simulink model "uz_6ph_pu_vsd_voltages_state_machine"  (R2021a)
settings: Solver=FixedStepDiscrete  StartTime=0.0  StopTime=3*t_ADC  RelTol=1e-3
values from neighbouring files (symbols this model uses):
  A = 1.0    (= 1)    [uz_6ph_pu_vsd_voltages_init.m]    (also in uz_mpc_6ph_init.m; uz_mpc_6ph_state_machine_init.m)
  f = n_rpm/60.0*p    (= 250)    [uz_6ph_pu_vsd_voltages_init.m]    (also in uz_mpc_6ph_init.m; uz_mpc_6ph_state_machine_init.m)
  t_ADC = 1/f_ADC    (= 1e-05)    [uz_6ph_pu_vsd_voltages_init.m]    (also in uz_mpc_6ph_init.m; uz_mpc_6ph_state_machine_init.m; uz_typeconv_init.m)
  t_clock = 1/f_clock    (= 1e-08)    [uz_6ph_pu_vsd_voltages_init.m]    (also in uz_mpc_6ph_init.m; uz_mpc_6ph_state_machine_init.m; uz_typeconv_init.m)
  v_dc = 565.0    (= 565)    [uz_6ph_pu_vsd_voltages_init.m]    (also in uz_mpc_6ph_init.m; uz_mpc_6ph_state_machine_init.m)
  VB = sqrt(2/3)*VR    [uz_6ph_pu_vsd_voltages_init.m]    (also in uz_mpc_6ph_init.m; uz_mpc_6ph_state_machine_init.m)
libraries: fl_lib x7, nesl_utility x7, simulink x3, hdlsllib x2, ee_lib x2
settings Model: DataTypeOverride=Off  Creator=micha  LastModifiedBy=micha
settings SolverCC: AlgebraicLoopSolver=TrustRegion
settings DataIOCC: LimitDataPoints=on  SaveOutput=off  SaveTime=off
settings OptimizationCC: BlockReduction=off  ConditionallyExecuteInputs=off  DefaultParameterBehavior=Inlined  LifeSpan=inf
settings DebuggingCC: AlgebraicLoopMsg=error  SingleTaskRateTransMsg=error  AllowSymbolicDim=off  StrictBusMsg=ErrorOnBusTreatedAsVector  SFUnexpectedBacktrackingDiag=warning  SFNoUnconditionalDefaultTransitionDiag=warning  SFExecutionAtInitializationDiag=none  SFMachineParentedDataDiag=warning  ArithmeticOperatorsInVariantConditions=warning
settings HardwareCC: ProdBitPerPointer=32  ProdBitPerSizeT=32  ProdBitPerPtrDiffT=32  ProdLargestAtomicFloat=None  ProdIntDivRoundTo=Undefined  ProdEndianess=Unspecified  ProdWordSize=32  ProdHWDeviceType=ASIC/FPGA->ASIC/FPGA  ProdEqTarget=off
settings SFSimCC: SimUseLocalCustomCode=off  CustomCodeUndefinedFunction=UseInterfaceOnly
settings RTWCC: RTWUseLocalCustomCode=off
settings CodeAppCC: StateflowObjectComments=on
settings GRTTargetCC: TargetLangStandard=C89/C90 (ANSI)
settings ConfigComp: CovScope=ReferencedModels  CovMetricSettings=dw  CovSaveCumulativeToWorkspaceVar=on  CovSaveSingleToWorkspaceVar=on  CovExternalEMLEnable=off  CovSFcnEnable=off

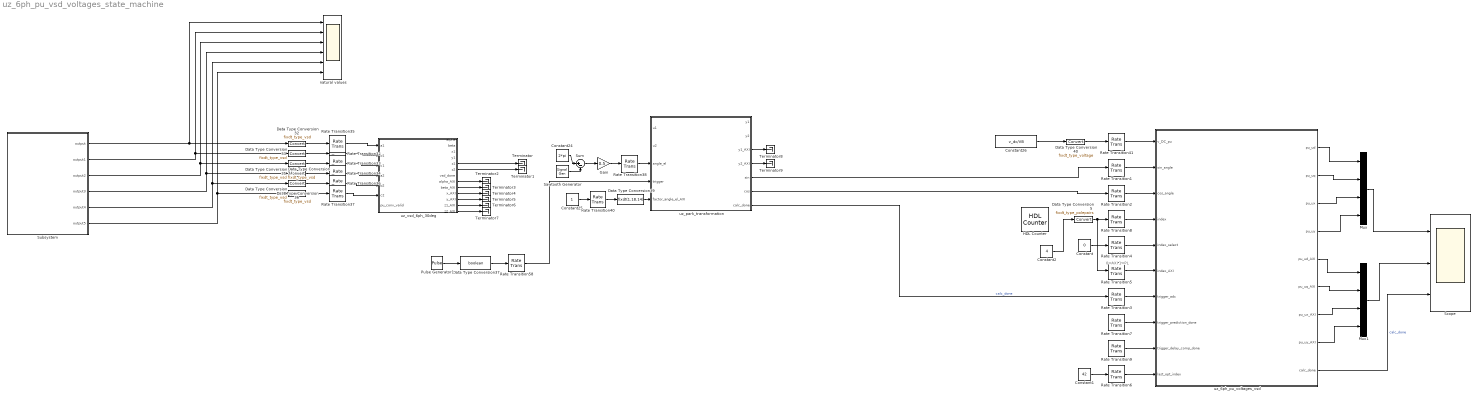
== system uz_6ph_pu_vsd_voltages_state_machine ==
  note: 0=AXI 1=PL
  Constant : Constant  Value=0  OutDataTypeStr=boolean
  Constant1 : Constant  Value=42  OutDataTypeStr=uint32
  Constant2 : Constant  Value=4  OutDataTypeStr=uint32
  Constant24 : Constant  Value=2*pi
  Constant25 : Constant
  Constant26 : Constant  Value=v_dc/VB
  Data Type Conversion{32..36,38} (6 alike) : DataTypeConversion  OutDataTypeStr=fixdt_type_vsd
  Data Type Conversion37 : DataTypeConversion  OutDataTypeStr=boolean
  Data Type Conversion39 : DataTypeConversion  OutDataTypeStr=fixdt(1,18,14)
  Data Type Conversion40 : DataTypeConversion  OutDataTypeStr=fixdt_type_voltage
  Data Type Conversion5 : DataTypeConversion  OutDataTypeStr=fixdt_type_polepairs
  Gain : Gain  Gain=0.5
  HDL Counter : hdlsllib/Sources/HDL Counter  CountType=Count limited  CountInit=1  CountStep=1  CountMax=64  CountFromType=Initial value  CountFrom=1  CountResetPort=off  CountLoadPort=off  CountEnbPort=off  CountDirPort=off  CountHitOutputPort=off  CountDataType=Unsigned  CountWordLen=8  CountFracLen=0  CountSampTime=t_ADC
  Mux : Mux
  Mux1 : Mux
  Pulse Generator1 : DiscretePulseGenerator  PulseType=Time based  Period=t_ADC  PulseWidth=5
  Rate Transition{1..2,4,32..38,40..41,58} (13 alike) : RateTransition  OutPortSampleTime=t_clock
  Rate Transition{3,5..9} (6 alike) : RateTransition  InitialCondition=1  OutPortSampleTime=t_clock
  Sawtooth Generator : SignalGenerator  WaveForm=sawtooth  Amplitude=2*pi  Frequency=2*pi*f  Units=rad/sec
  Scope : Scope  NumInputPorts=3
  Subsystem : Subsystem
  Sum : Sum  Inputs=|+-
  Terminator{,1..9} (10 alike) : Terminator
  natural values : Scope  NumInputPorts=6
  uz_6ph_pu_voltages_vsd : Subsystem  TreatAsAtomicUnit=on
  uz_park_transformation : Subsystem  TreatAsAtomicUnit=on
  uz_vsd_6ph_30deg : Subsystem  TreatAsAtomicUnit=on
  wires:
  Data Type Conversion5/1 -> Rate Transition8/1, Rate Transition5/1
  Rate Transition8/1 -> uz_6ph_pu_voltages_vsd/4(index)
  Constant26/1 -> Data Type Conversion40/1
  Rate Transition41/1 -> uz_6ph_pu_voltages_vsd/1(v_DC_pu)
  Data Type Conversion40/1 -> Rate Transition41/1
  Data Type Conversion35/1 -> Rate Transition34/1
  uz_vsd_6ph_30deg/5(z1) -> Terminator/1
  Rate Transition40/1 -> Data Type Conversion39/1
  Sawtooth Generator/1 -> Sum/2
  Constant25/1 -> Rate Transition40/1
  Data Type Conversion34/1 -> Rate Transition33/1
  Gain/1 -> Rate Transition38/1
  Subsystem/4(output3) -> Data Type Conversion35/1, natural values/4
  Sum/1 -> Gain/1
  Subsystem/5(output4) -> Data Type Conversion36/1, natural values/5
  Rate Transition33/1 -> uz_vsd_6ph_30deg/3(c1)
  uz_vsd_6ph_30deg/9(beta_AXI) -> Terminator3/1
  Rate Transition34/1 -> uz_vsd_6ph_30deg/4(a2)
  Rate Transition37/1 -> uz_vsd_6ph_30deg/6(c2)
  uz_vsd_6ph_30deg/6(z2) -> Terminator1/1
  uz_vsd_6ph_30deg/10(x_AXI) -> Terminator4/1
  Data Type Conversion39/1 -> uz_park_transformation/5(factor_angle_el_AXI)
  Subsystem/3(output2) -> Data Type Conversion34/1, natural values/3
  Subsystem/2(output1) -> natural values/2, Data Type Conversion33/1
  Data Type Conversion38/1 -> Rate Transition37/1
  Data Type Conversion33/1 -> Rate Transition32/1
  Rate Transition35/1 -> uz_vsd_6ph_30deg/1(a1)
  Rate Transition36/1 -> uz_vsd_6ph_30deg/5(b2)
  Constant24/1 -> Sum/1
  Subsystem/1(output) -> natural values/1, Data Type Conversion32/1
  uz_vsd_6ph_30deg/11(y_AXI) -> Terminator5/1
  Subsystem/6(output5) -> natural values/6, Data Type Conversion38/1
  uz_park_transformation/3(y1_AXI) -> Terminator8/1
  Rate Transition32/1 -> uz_vsd_6ph_30deg/2(b1)
  uz_vsd_6ph_30deg/8(alpha_AXI) -> Terminator2/1
  Data Type Conversion36/1 -> Rate Transition36/1
  uz_vsd_6ph_30deg/12(z1_AXI) -> Terminator6/1
  uz_park_transformation/4(y2_AXI) -> Terminator9/1
  Data Type Conversion32/1 -> Rate Transition35/1
  uz_vsd_6ph_30deg/13(z2_AXI) -> Terminator7/1
  uz_park_transformation/5(sin) -> Rate Transition1/1
  uz_park_transformation/6(cos) -> Rate Transition2/1
  Rate Transition1/1 -> uz_6ph_pu_voltages_vsd/2(sin_angle)
  Rate Transition2/1 -> uz_6ph_pu_voltages_vsd/3(cos_angle)
  Data Type Conversion37/1 -> Rate Transition58/1
  Rate Transition58/1 -> uz_park_transformation/4(trigger)
  Pulse Generator1/1 -> Data Type Conversion37/1
  Rate Transition3/1 -> uz_6ph_pu_voltages_vsd/7(trigger_adc)
  uz_park_transformation/7(calc_done) -> Rate Transition3/1  "calc_done"
  uz_6ph_pu_voltages_vsd/1(pu_ud) -> Mux/1
  uz_6ph_pu_voltages_vsd/2(pu_uq) -> Mux/2
  uz_6ph_pu_voltages_vsd/3(pu_ux) -> Mux/3
  uz_6ph_pu_voltages_vsd/4(pu_uy) -> Mux/4
  Mux/1 -> Scope/1
  uz_6ph_pu_voltages_vsd/9(calc_done) -> Scope/3  "calc_done"
  Constant2/1 -> Data Type Conversion5/1
  Rate Transition38/1 -> uz_park_transformation/3(angle_el)
  Rate Transition4/1 -> uz_6ph_pu_voltages_vsd/5(index_select)
  Rate Transition5/1 -> uz_6ph_pu_voltages_vsd/6(index_AXI)
  Constant/1 -> Rate Transition4/1
  Mux1/1 -> Scope/2
  uz_6ph_pu_voltages_vsd/5(pu_ud_AXI) -> Mux1/1
  uz_6ph_pu_voltages_vsd/8(pu_uy_AXI) -> Mux1/4
  uz_6ph_pu_voltages_vsd/7(pu_ux_AXI) -> Mux1/3
  uz_6ph_pu_voltages_vsd/6(pu_uq_AXI) -> Mux1/2
  Rate Transition6/1 -> uz_6ph_pu_voltages_vsd/10(last_opt_index)
  Constant1/1 -> Rate Transition6/1
  Rate Transition7/1 -> uz_6ph_pu_voltages_vsd/8(trigger_prediction_done)
  Rate Transition9/1 -> uz_6ph_pu_voltages_vsd/9(trigger_delay_comp_done)

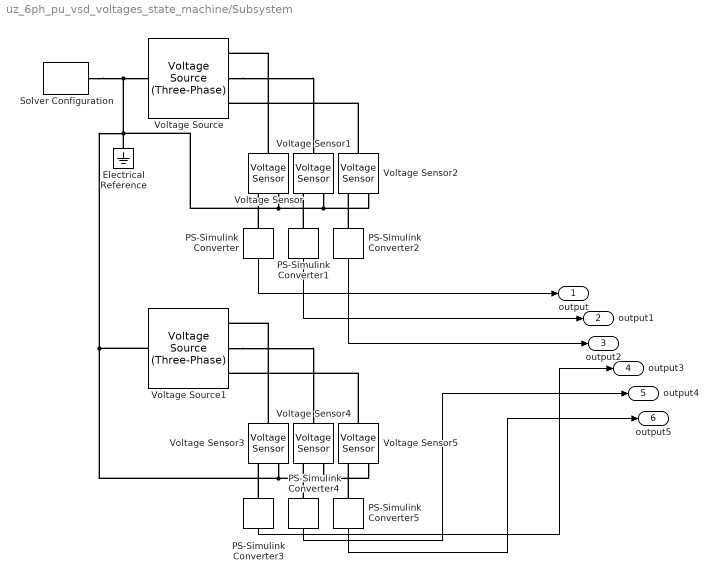
== system uz_6ph_pu_vsd_voltages_state_machine/Subsystem ==
  Electrical Reference : fl_lib/Electrical/Electrical Elements/Electrical Reference
  PS-Simulink Converter{,1..5} (6 alike) : nesl_utility/PS-Simulink Converter  PhysicalDomain=network_engine_domain  SubClassName=ps_output  LeftPortType=input  RightPortType=output  PseudoPeriodic=off  Frequencies=[]  Unit=1  AffineConversion=off
  Solver Configuration : nesl_utility/Solver Configuration  PhysicalDomain=network_engine_domain  SubClassName=solver  LeftPortType=input  RightPortType=generic  Tones=[]  Harmonics=[]  SimulateNoise=off  Profile=off  UseLocalSampling=off  EnableSwitchedLinearOptims=on  FrequencyDomain=off  UseCCode=off  RelTol=0.001  AbsTol=1e-06  MinStep=1e-09  ToWorkspace=off  RevertToSquareIcSolve=off  NumHomotopyIterations=100  PhasorMode=off  PhasorModeNumHarmonics=1  DoDC=off  ResidualTolerance=1e-09  UseLocalSolver=on  LocalSolverChoice=NE_BACKWARD_EULER_ADVANCER  LocalSolverSampleTime=1e-6  DoFixedCost=on  MaxNonlinIter=3  MaxModeIter=2  ComputeImpulses=off  ImpulseIterations=2  LinearAlgebra=Sparse  EquationFormulation=NE_TIME_EF  DelaysMemoryBudget=1024  AutomaticFiltering=on  FilteringTimeConstant=0.001  PartitionStorageMethod=AS_NEEDED  PartitionMemoryBudget=1024  PartitionMethod=FAST
  Voltage Sensor{,1..5} (6 alike) : fl_lib/Electrical/Electrical Sensors/Voltage Sensor
  Voltage Source : ee_lib/Sources/Voltage Source (Three-Phase)  vline_rms=A*sqrt(3)/sqrt(2) V  shift=0 deg  freq=f Hz  impedance_option=1  SShortCircuit=1e6 V*A  XR=15  R=0.01 Ohm  L=3.97e-4 H  G_parasitic=0 1/Ohm  harmonic_option=1  harmonic_orders=Harmonic_Orders  harmonic_ratios=Harmonic_Amplitudes  I_specify=off  I_priority=None  I=[ 0 0 0 ] A  I_nominal_specify=off  I_nominal_unit=A  I_nominal_value=1
      settings: SourceProductBaseCode=PS  InternalSimscapePortConfiguration="{\"Bottom\":[],\"Left\":[{\"id\":\"n\",\"label\":\"n\",\"type\":\"foundation.electrical.electrical\"}],\"Right\":[{\"id\":\"a\",\"label\":\"a\",\"type\":\"foundation.electrical.electrical\"},{\"id\":\"b\",\"label\":\"b\",\"type\":\"foundation.electrical.electrical\"},{\"id\":\"c\",\"label\":\"c\",\"type\":\"foundation.electrical.electrical\"}],\"Top\":[]}"
  Voltage Source1 : ee_lib/Sources/Voltage Source (Three-Phase)  vline_rms=A*sqrt(3)/sqrt(2) V  shift=-30 deg  freq=f Hz  impedance_option=1  SShortCircuit=1e6 V*A  XR=15  R=0.01 Ohm  L=3.97e-4 H  G_parasitic=0 1/Ohm  harmonic_option=1  harmonic_orders=Harmonic_Orders  harmonic_ratios=Harmonic_Amplitudes  I_specify=off  I_priority=None  I=[ 0 0 0 ] A  I_nominal_specify=off  I_nominal_unit=A  I_nominal_value=1
      settings: SourceProductBaseCode=PS  InternalSimscapePortConfiguration="{\"Bottom\":[],\"Left\":[{\"id\":\"n\",\"label\":\"n\",\"type\":\"foundation.electrical.electrical\"}],\"Right\":[{\"id\":\"a\",\"label\":\"a\",\"type\":\"foundation.electrical.electrical\"},{\"id\":\"b\",\"label\":\"b\",\"type\":\"foundation.electrical.electrical\"},{\"id\":\"c\",\"label\":\"c\",\"type\":\"foundation.electrical.electrical\"}],\"Top\":[]}"
  output : Outport
  output1 : Outport  Port=2
  output2 : Outport  Port=3
  output3 : Outport  Port=4
  output4 : Outport  Port=5
  output5 : Outport  Port=6
  wires:
  PS-Simulink Converter/1 -> output/1
  PS-Simulink Converter3/1 -> output3/1
  PS-Simulink Converter4/1 -> output4/1
  PS-Simulink Converter1/1 -> output1/1
  PS-Simulink Converter5/1 -> output5/1
  PS-Simulink Converter2/1 -> output2/1
  connections:
  Voltage Sensor5/RConn2 -- Solver Configuration/RConn1 -- Voltage Source/LConn1 -- Voltage Sensor2/RConn2 -- Voltage Sensor1/RConn2 -- Voltage Sensor/RConn2 -- Electrical Reference/LConn1 -- Voltage Source1/LConn1 -- Voltage Sensor3/RConn2 -- Voltage Sensor4/RConn2
  PS-Simulink Converter5/LConn1 -- Voltage Sensor5/RConn1
  PS-Simulink Converter1/LConn1 -- Voltage Sensor1/RConn1
  Voltage Sensor3/LConn1 -- Voltage Source1/RConn1
  PS-Simulink Converter/LConn1 -- Voltage Sensor/RConn1
  Voltage Source1/RConn2 -- Voltage Sensor4/LConn1
  Voltage Sensor5/LConn1 -- Voltage Source1/RConn3
  PS-Simulink Converter4/LConn1 -- Voltage Sensor4/RConn1
  Voltage Sensor2/LConn1 -- Voltage Source/RConn3
  PS-Simulink Converter2/LConn1 -- Voltage Sensor2/RConn1
  PS-Simulink Converter3/LConn1 -- Voltage Sensor3/RConn1
  Voltage Sensor/LConn1 -- Voltage Source/RConn1
  Voltage Source/RConn2 -- Voltage Sensor1/LConn1

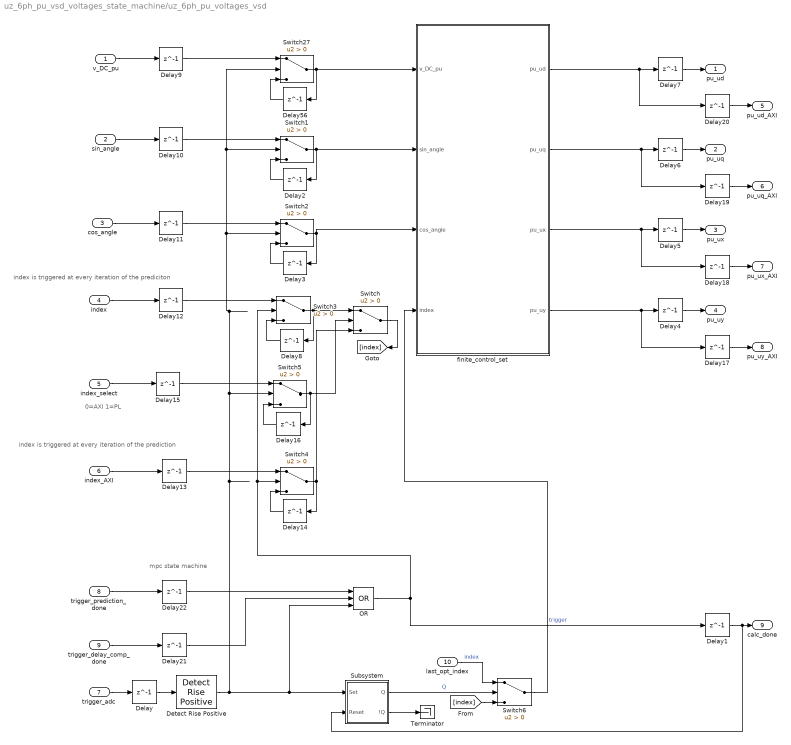
== system uz_6ph_pu_vsd_voltages_state_machine/uz_6ph_pu_voltages_vsd ==
  note: index is triggered at every iteration of the prediction
  note: index is triggered at every iteration of the prediciton
  note: 0=AXI 1=PL
  note: mpc state machine
  v_DC_pu : Inport  OutDataTypeStr=fixdt_type_constants
  sin_angle : Inport  Port=2  OutDataTypeStr=fixdt_type_sin_cos
  cos_angle : Inport  Port=3  OutDataTypeStr=fixdt_type_sin_cos
  index : Inport  Port=4
  index_select : Inport  Port=5
  index_AXI : Inport  Port=6
  trigger_adc : Inport  Port=7
  trigger_prediction_done : Inport  Port=8
  trigger_delay_comp_done : Inport  Port=9
  last_opt_index : Inport  Port=10
  Delay{,1..7,9..13,15,17..22,56} (21 alike) : Delay  DelayLength=1
  Delay14 : Delay  DelayLength=1  InitialCondition=1
  Delay16 : Delay  DelayLength=1  InitialCondition=1
  Delay8 : Delay  DelayLength=1  InitialCondition=1
  Detect Rise Positive : simulink/Logic and Bit Operations/Detect Rise Positive  vinit=0  OutDataTypeStr=boolean
  OR : Logic  Operator=OR  Inputs=3  IconShape=distinctive  AllPortsSameDT=off  OutDataTypeStr=boolean
  Subsystem : Subsystem
  Switch : Switch  Criteria=u2 > Threshold
  Switch1 : Switch  Criteria=u2 > Threshold  OutDataTypeStr=fixdt_type_sin_cos
  Switch2 : Switch  Criteria=u2 > Threshold  OutDataTypeStr=fixdt_type_sin_cos
  Switch27 : Switch  Criteria=u2 > Threshold  OutDataTypeStr=fixdt_type_constants
  Switch3 : Switch  Criteria=u2 > Threshold  OutDataTypeStr=fixdt_type_polepairs
  Switch4 : Switch  Criteria=u2 > Threshold  OutDataTypeStr=fixdt_type_polepairs
  Switch5 : Switch  Criteria=u2 > Threshold  OutDataTypeStr=fixdt_type_polepairs
  Switch6 : Switch  Criteria=u2 > Threshold
  Terminator : Terminator
  finite_control_set : MATLAB Function  TreatAsAtomicUnit=on
  pu_ud : Outport
  pu_uq : Outport  Port=2
  pu_ux : Outport  Port=3
  pu_uy : Outport  Port=4
  pu_ud_AXI : Outport  Port=5
  pu_uq_AXI : Outport  Port=6
  pu_ux_AXI : Outport  Port=7
  pu_uy_AXI : Outport  Port=8
  calc_done : Outport  Port=9
  wires:
  finite_control_set/1(pu_ud) -> Delay20/1, Delay7/1
  finite_control_set/2(pu_uq) -> Delay19/1, Delay6/1
  finite_control_set/3(pu_ux) -> Delay18/1, Delay5/1
  finite_control_set/4(pu_uy) -> Delay17/1, Delay4/1
  trigger_adc/1 -> Delay/1
  Delay/1 -> Detect Rise Positive/1
  Delay56/1 -> Switch27/3
  v_DC_pu/1 -> Delay9/1
  Switch27/1 -> Delay56/1, finite_control_set/1(v_DC_pu)
  sin_angle/1 -> Delay10/1
  Delay2/1 -> Switch1/3
  Switch1/1 -> finite_control_set/2(sin_angle), Delay2/1
  cos_angle/1 -> Delay11/1
  Delay3/1 -> Switch2/3
  Switch2/1 -> finite_control_set/3(cos_angle), Delay3/1
  Delay4/1 -> pu_uy/1
  Delay5/1 -> pu_ux/1
  Delay6/1 -> pu_uq/1
  Delay7/1 -> pu_ud/1
  Switch3/1 -> Delay8/1, Switch/1
  index/1 -> Delay12/1
  Delay8/1 -> Switch3/3
  Delay9/1 -> Switch27/1
  Delay10/1 -> Switch1/1
  Delay11/1 -> Switch2/1
  Delay12/1 -> Switch3/1
  Delay14/1 -> Switch4/3
  index_AXI/1 -> Delay13/1
  Switch4/1 -> Switch/3, Delay14/1
  Delay13/1 -> Switch4/1
  Delay16/1 -> Switch5/3
  index_select/1 -> Delay15/1
  Switch5/1 -> Switch/2, Delay16/1
  Delay15/1 -> Switch5/1
  Delay17/1 -> pu_uy_AXI/1
  Delay19/1 -> pu_uq_AXI/1
  Delay20/1 -> pu_ud_AXI/1
  Delay18/1 -> pu_ux_AXI/1
  trigger_prediction_done/1 -> Delay22/1
  trigger_delay_comp_done/1 -> Delay21/1
  Delay21/1 -> OR/2
  OR/1 -> Switch3/2, Switch4/2, Delay1/1  "trigger"
  Delay22/1 -> OR/1
  Detect Rise Positive/1 -> Subsystem/1(Set), OR/3, Switch5/2, Switch2/2, Switch1/2, Switch27/2
  Subsystem/2(!Q) -> Terminator/1
  Delay1/1 -> Subsystem/2(Reset), calc_done/1
  Subsystem/1(Q) -> Switch6/2  "Q"
  last_opt_index/1 -> Switch6/1  "index"
  Switch/1 -> [index]
  [index] -> Switch6/3
  Switch6/1 -> finite_control_set/4(index)

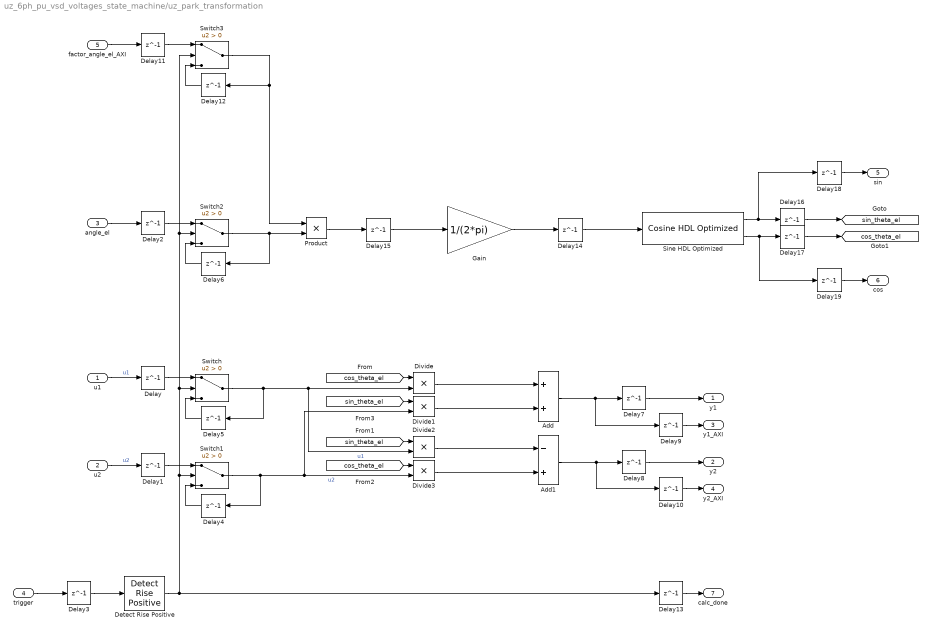
== system uz_6ph_pu_vsd_voltages_state_machine/uz_park_transformation ==
  u1 : Inport
  u2 : Inport  Port=2
  angle_el : Inport  Port=3
  trigger : Inport  Port=4
  factor_angle_el_AXI : Inport  Port=5
  Add : Sum  OutDataTypeStr=fixdt(1,27,16)
  Add1 : Sum  Inputs=-+  OutDataTypeStr=fixdt(1,27,16)
  Delay{,1..19} (20 alike) : Delay  DelayLength=1
  Detect Rise Positive : simulink/Logic and Bit Operations/Detect Rise Positive  vinit=0  OutDataTypeStr=boolean
  Divide{,1..3} (4 alike) : Product  Inputs=**  OutDataTypeStr=fixdt(1,27,16)
  Gain : Gain  Gain=1/(2*pi)  OutDataTypeStr=fixdt(1,18,16)
  Product : Product  OutDataTypeStr=fixdt(1,18,14)
  Sine HDL Optimized : hdlsllib/Lookup Tables/Cosine HDL Optimized  OutputFormula=sin(2*pi*u) and cos(2*pi*u)  NumDataPoints=256  TableDataTypeStr=fixdt(0,17,16)  SimulateLUTROMDelay=off
      settings: SourceProductBaseCode=SL
  Switch{,1..3} (4 alike) : Switch  Criteria=u2 > Threshold
  y1 : Outport  VectorParamsAs1DForOutWhenUnconnected=off
  y2 : Outport  Port=2  VectorParamsAs1DForOutWhenUnconnected=off
  y1_AXI : Outport  Port=3  VectorParamsAs1DForOutWhenUnconnected=off
  y2_AXI : Outport  Port=4  VectorParamsAs1DForOutWhenUnconnected=off
  sin : Outport  Port=5  VectorParamsAs1DForOutWhenUnconnected=off
  cos : Outport  Port=6  VectorParamsAs1DForOutWhenUnconnected=off
  calc_done : Outport  Port=7  VectorParamsAs1DForOutWhenUnconnected=off
  tag scope: cos_theta_el=global, sin_theta_el=global
  wires:
  Switch1/1 -> Delay4/1, Divide1/2, Divide3/2  "u2"
  Divide2/1 -> Add1/1
  Divide3/1 -> Add1/2
  [cos_theta_el] -> Divide3/1
  Switch/1 -> Divide2/2, Divide/2, Delay5/1  "u1"
  [sin_theta_el] -> Divide2/1
  Divide1/1 -> Add/2
  [cos_theta_el] -> Divide/1
  [sin_theta_el] -> Divide1/1
  Add/1 -> Delay9/1, Delay7/1
  Add1/1 -> Delay10/1, Delay8/1
  Divide/1 -> Add/1
  angle_el/1 -> Delay2/1
  Sine HDL Optimized/2 -> Delay19/1, Delay17/1
  Sine HDL Optimized/1 -> Delay18/1, Delay16/1
  Gain/1 -> Delay14/1
  u1/1 -> Delay/1  "u1"
  u2/1 -> Delay1/1  "u2"
  Delay/1 -> Switch/1
  Delay1/1 -> Switch1/1
  Delay2/1 -> Switch2/1
  trigger/1 -> Delay3/1
  Delay4/1 -> Switch1/3
  Delay5/1 -> Switch/3
  Delay6/1 -> Switch2/3
  Delay7/1 -> y1/1
  Delay8/1 -> y2/1
  Delay9/1 -> y1_AXI/1
  Delay10/1 -> y2_AXI/1
  Switch2/1 -> Product/2, Delay6/1
  Switch3/1 -> Product/1, Delay12/1
  factor_angle_el_AXI/1 -> Delay11/1
  Detect Rise Positive/1 -> Delay13/1, Switch1/2, Switch/2, Switch3/2, Switch2/2
  Delay12/1 -> Switch3/3
  Delay11/1 -> Switch3/1
  Product/1 -> Delay15/1
  Delay3/1 -> Detect Rise Positive/1
  Delay13/1 -> calc_done/1
  Delay15/1 -> Gain/1
  Delay14/1 -> Sine HDL Optimized/1
  Delay16/1 -> [sin_theta_el]
  Delay17/1 -> [cos_theta_el]
  Delay18/1 -> sin/1
  Delay19/1 -> cos/1

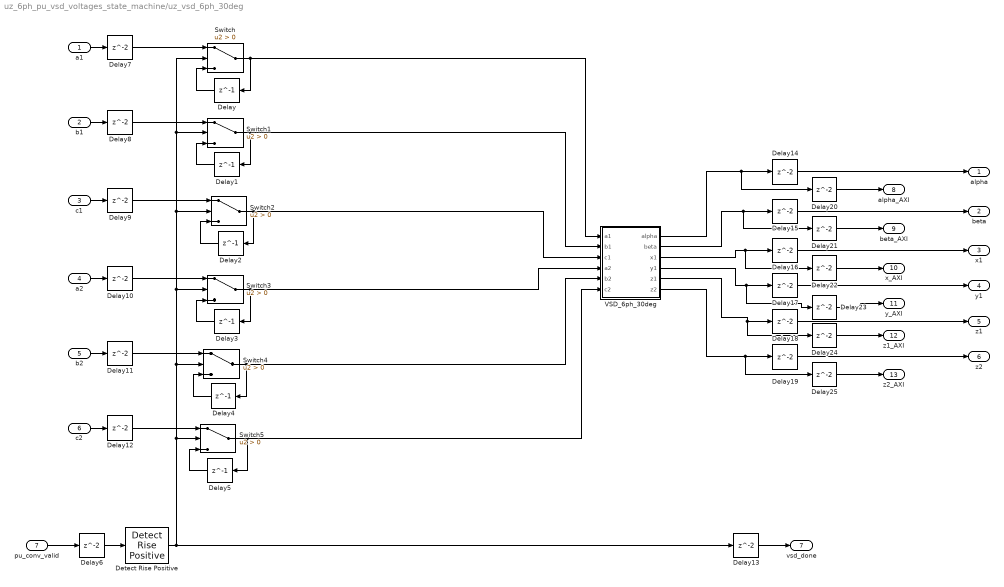
== system uz_6ph_pu_vsd_voltages_state_machine/uz_vsd_6ph_30deg ==
  a1 : Inport
  b1 : Inport  Port=2
  c1 : Inport  Port=3
  a2 : Inport  Port=4
  b2 : Inport  Port=5
  c2 : Inport  Port=6
  pu_conv_valid : Inport  Port=7
  Delay{,1..5} (6 alike) : Delay  DelayLength=1
  Delay{6..25} (20 alike) : Delay
  Detect Rise Positive : simulink/Logic and Bit Operations/Detect Rise Positive  vinit=0  OutDataTypeStr=boolean
  Switch{,1..5} (6 alike) : Switch  Criteria=u2 > Threshold  OutDataTypeStr=fixdt_type_vsd
  VSD_6ph_30deg : MATLAB Function  TreatAsAtomicUnit=on
  alpha : Outport  OutDataTypeStr=fixdt(1,18,11)  VectorParamsAs1DForOutWhenUnconnected=off
  beta : Outport  Port=2  OutDataTypeStr=fixdt(1,18,11)  VectorParamsAs1DForOutWhenUnconnected=off
  x1 : Outport  Port=3  OutDataTypeStr=fixdt(1,18,11)  VectorParamsAs1DForOutWhenUnconnected=off
  y1 : Outport  Port=4  OutDataTypeStr=fixdt(1,18,11)  VectorParamsAs1DForOutWhenUnconnected=off
  z1 : Outport  Port=5  OutDataTypeStr=fixdt(1,18,11)  VectorParamsAs1DForOutWhenUnconnected=off
  z2 : Outport  Port=6  OutDataTypeStr=fixdt(1,18,11)  VectorParamsAs1DForOutWhenUnconnected=off
  vsd_done : Outport  Port=7  VectorParamsAs1DForOutWhenUnconnected=off
  alpha_AXI : Outport  Port=8  OutDataTypeStr=fixdt(1,18,11)  VectorParamsAs1DForOutWhenUnconnected=off
  beta_AXI : Outport  Port=9  OutDataTypeStr=fixdt(1,18,11)  VectorParamsAs1DForOutWhenUnconnected=off
  x_AXI : Outport  Port=10  OutDataTypeStr=fixdt(1,18,11)  VectorParamsAs1DForOutWhenUnconnected=off
  y_AXI : Outport  Port=11  OutDataTypeStr=fixdt(1,18,11)  VectorParamsAs1DForOutWhenUnconnected=off
  z1_AXI : Outport  Port=12  OutDataTypeStr=fixdt(1,18,11)  VectorParamsAs1DForOutWhenUnconnected=off
  z2_AXI : Outport  Port=13  OutDataTypeStr=fixdt(1,18,11)  VectorParamsAs1DForOutWhenUnconnected=off
  wires:
  VSD_6ph_30deg/1(alpha) -> Delay20/1, Delay14/1
  VSD_6ph_30deg/2(beta) -> Delay21/1, Delay15/1
  VSD_6ph_30deg/3(x1) -> Delay22/1, Delay16/1
  VSD_6ph_30deg/4(y1) -> Delay23/1, Delay17/1
  VSD_6ph_30deg/5(z1) -> Delay24/1, Delay18/1
  VSD_6ph_30deg/6(z2) -> Delay25/1, Delay19/1
  pu_conv_valid/1 -> Delay6/1
  Detect Rise Positive/1 -> Switch5/2, Switch4/2, Switch3/2, Switch2/2, Switch1/2, Switch/2, Delay13/1
  Delay/1 -> Switch/3
  Switch/1 -> VSD_6ph_30deg/1(a1), Delay/1
  Delay1/1 -> Switch1/3
  Switch1/1 -> VSD_6ph_30deg/2(b1), Delay1/1
  Delay2/1 -> Switch2/3
  Switch2/1 -> VSD_6ph_30deg/3(c1), Delay2/1
  Delay3/1 -> Switch3/3
  Switch3/1 -> VSD_6ph_30deg/4(a2), Delay3/1
  Delay4/1 -> Switch4/3
  Switch4/1 -> VSD_6ph_30deg/5(b2), Delay4/1
  Delay5/1 -> Switch5/3
  Switch5/1 -> VSD_6ph_30deg/6(c2), Delay5/1
  a1/1 -> Delay7/1
  b1/1 -> Delay8/1
  c1/1 -> Delay9/1
  a2/1 -> Delay10/1
  b2/1 -> Delay11/1
  c2/1 -> Delay12/1
  Delay6/1 -> Detect Rise Positive/1
  Delay7/1 -> Switch/1
  Delay8/1 -> Switch1/1
  Delay9/1 -> Switch2/1
  Delay10/1 -> Switch3/1
  Delay11/1 -> Switch4/1
  Delay12/1 -> Switch5/1
  Delay13/1 -> vsd_done/1
  Delay14/1 -> alpha/1
  Delay15/1 -> beta/1
  Delay16/1 -> x1/1
  Delay17/1 -> y1/1
  Delay18/1 -> z1/1
  Delay19/1 -> z2/1
  Delay20/1 -> alpha_AXI/1
  Delay21/1 -> beta_AXI/1
  Delay22/1 -> x_AXI/1
  Delay23/1 -> y_AXI/1
  Delay24/1 -> z1_AXI/1
  Delay25/1 -> z2_AXI/1

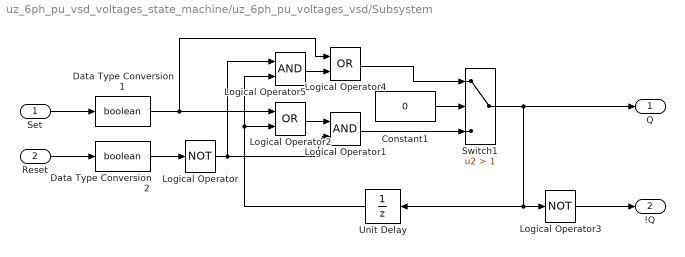
== system uz_6ph_pu_vsd_voltages_state_machine/uz_6ph_pu_voltages_vsd/Subsystem ==
  Set : Inport
  Reset : Inport  Port=2
  Constant1 : Constant  Value=0  OutDataTypeStr=uint32  SampleTime=-1
  Data Type Conversion1 : DataTypeConversion  OutDataTypeStr=boolean
  Data Type Conversion2 : DataTypeConversion  OutDataTypeStr=boolean
  Logical Operator : Logic  Operator=NOT  AllPortsSameDT=off  OutDataTypeStr=boolean
  Logical Operator1 : Logic  AllPortsSameDT=off  OutDataTypeStr=boolean
  Logical Operator2 : Logic  Operator=OR  AllPortsSameDT=off  OutDataTypeStr=boolean
  Logical Operator3 : Logic  Operator=NOT  AllPortsSameDT=off  OutDataTypeStr=boolean
  Logical Operator4 : Logic  Operator=OR  AllPortsSameDT=off  OutDataTypeStr=boolean
  Logical Operator5 : Logic  AllPortsSameDT=off  OutDataTypeStr=boolean
  Switch1 : Switch  Criteria=u2 > Threshold  Threshold=1
  Unit Delay : UnitDelay  SampleTime=t_clock  HasFrameUpgradeWarning=on
  Q : Outport  VectorParamsAs1DForOutWhenUnconnected=off
  !Q : Outport  Port=2  VectorParamsAs1DForOutWhenUnconnected=off
  wires:
  Logical Operator/1 -> Logical Operator1/2, Logical Operator5/1
  Reset/1 -> Data Type Conversion2/1
  Constant1/1 -> Switch1/2
  Logical Operator4/1 -> Switch1/1
  Data Type Conversion1/1 -> Logical Operator2/1, Logical Operator4/1
  Switch1/1 -> Q/1, Unit Delay/1, Logical Operator3/1
  Logical Operator3/1 -> !Q/1
  Set/1 -> Data Type Conversion1/1
  Logical Operator2/1 -> Logical Operator1/1
  Unit Delay/1 -> Logical Operator2/2, Logical Operator5/2
  Logical Operator5/1 -> Logical Operator4/2
  Logical Operator1/1 -> Switch1/3
  Data Type Conversion2/1 -> Logical Operator/1

== matlab function uz_6ph_pu_vsd_voltages_state_machine/uz_vsd_6ph_30deg/VSD_6ph_30deg ==
  settings: fimath=fimath('RoundingMethod', 'Floor','OverflowAction', 'Wrap','ProductMode', 'FullPrecision', 'SumMode', 'FullPrecision')
  data: a1 input; alpha output; b1 input; c1 input; a2 input; b2 input; c2 input; beta output; x1 output; y1 output; z1 output; z2 output
function [alpha,beta,x1,y1,z1,z2] = fcn(a1,b1,c1,a2,b2,c2)


A = [fi(0,1,18,11) fi(0,1,18,11) fi(0,1,18,11) fi(0,1,18,11) fi(0,1,18,11) fi(0,1,18,11)]';

A =    2/6*[1    -0.5        -0.5        sqrt(3)/2   -sqrt(3)/2  0 ;
           0    sqrt(3)/2   -sqrt(3)/2  0.5         0.5         -1;
           1    -0.5        -0.5        -sqrt(3)/2  sqrt(3)/2   0 ;
           0    -sqrt(3)/2  sqrt(3)/2   0.5         0.5         -1;
           0.5   0.5          0.5          0           0           0 ;
           0    0           0           0.5          0.5          0.5] * [a1 b1 c1 a2 b2 c2]';

alpha = fi(A(1),1,18,11);
beta = fi(A(2),1,18,11);
x1 = fi(A(3),1,18,11);
y1 = fi(A(4),1,18,11);
z1 = fi(A(5),1,18,11);
z2 = fi(A(6),1,18,11);

== matlab function uz_6ph_pu_vsd_voltages_state_machine/uz_6ph_pu_voltages_vsd/finite_control_set ==
  settings: fimath=fimath('RoundingMethod', 'Floor','OverflowAction', 'Wrap','ProductMode', 'FullPrecision', 'SumMode', 'FullPrecision')
  data: v_DC_pu input; sin_angle input; pu_ud output; pu_uq output; pu_ux output; pu_uy output; cos_angle input; index input
function [pu_ud,pu_uq,pu_ux,pu_uy] = voltage_space_vectors(v_DC_pu, sin_angle, cos_angle, index)

fm = fimath();
v_DC_pu = fi(v_DC_pu,1,18,15,fm);
sin_angle = fi(sin_angle,1,18,16,fm);
cos_angle = fi(cos_angle,1,18,16,fm);

% u_d-voltages lookup factors alpha/beta
vd_pu = fi([0.000000,  0.000000;
0.333333,  -0.000000;
-0.166667,  0.288675;
0.166667,  0.288675;
-0.166667,  -0.288675;
0.166667,  -0.288675;
-0.333333,  0.000000;
0.000000,  0.000000;
0.288675,  0.166667;
0.622008,  0.166667;
0.122008,  0.455342;
0.455342,  0.455342;
0.122008,  -0.122008;
0.455342,  -0.122008;
-0.044658,  0.166667;
0.288675,  0.166667;
-0.288675,  0.166667;
0.044658,  0.166667;
-0.455342,  0.455342;
-0.122008,  0.455342;
-0.455342,  -0.122008;
-0.122008,  -0.122008;
-0.622008,  0.166667;
-0.288675,  0.166667;
0.000000,  0.333333;
0.333333,  0.333333;
-0.166667,  0.622008;
0.166667,  0.622008;
-0.166667,  0.044658;
0.166667,  0.044658;
-0.333333,  0.333333;
0.000000,  0.333333;
-0.000000,  -0.333333;
0.333333,  -0.333333;
-0.166667,  -0.044658;
0.166667,  -0.044658;
-0.166667,  -0.622008;
0.166667,  -0.622008;
-0.333333,  -0.333333;
-0.000000,  -0.333333;
0.288675,  -0.166667;
0.622008,  -0.166667;
0.122008,  0.122008;
0.455342,  0.122008;
0.122008,  -0.455342;
0.455342,  -0.455342;
-0.044658,  -0.166667;
0.288675,  -0.166667;
-0.288675,  -0.166667;
0.044658,  -0.166667;
-0.455342,  0.122008;
-0.122008,  0.122008;
-0.455342,  -0.455342;
-0.122008,  -0.455342;
-0.622008,  -0.166667;
-0.288675,  -0.166667;
0.000000,  0.000000;
0.333333,  -0.000000;
-0.166667,  0.288675;
0.166667,  0.288675;
-0.166667,  -0.288675;
0.166667,  -0.288675;
-0.333333,  0.000000;
0.000000,  0.000000],1,18,15);

% u_q-voltages lookup factors alpha/beta
vq_pu = fi([0.000000, 0.000000;
0.333333, -0.000000;
-0.166667, 0.288675;
0.166667, 0.288675;
-0.166667, -0.288675;
0.166667, -0.288675;
-0.333333, 0.000000;
0.000000, 0.000000;
0.288675, 0.166667;
0.622008, 0.166667;
0.122008, 0.455342;
0.455342, 0.455342;
0.122008, -0.122008;
0.455342, -0.122008;
-0.044658, 0.166667;
0.288675, 0.166667;
-0.288675, 0.166667;
0.044658, 0.166667;
-0.455342, 0.455342;
-0.122008, 0.455342;
-0.455342, -0.122008;
-0.122008, -0.122008;
-0.622008, 0.166667;
-0.288675, 0.166667;
0.000000, 0.333333;
0.333333, 0.333333;
-0.166667, 0.622008;
0.166667, 0.622008;
-0.166667, 0.044658;
0.166667, 0.044658;
-0.333333, 0.333333;
0.000000, 0.333333;
-0.000000, -0.333333;
0.333333, -0.333333;
-0.166667, -0.044658;
0.166667, -0.044658;
-0.166667, -0.622008;
0.166667, -0.622008;
-0.333333, -0.333333;
-0.000000, -0.333333;
0.288675, -0.166667;
0.622008, -0.166667;
0.122008, 0.122008;
0.455342, 0.122008;
0.122008, -0.455342;
0.455342, -0.455342;
-0.044658, -0.166667;
0.288675, -0.166667;
-0.288675, -0.166667;
0.044658, -0.166667;
-0.455342, 0.122008;
-0.122008, 0.122008;
-0.455342, -0.455342;
-0.122008, -0.455342;
-0.622008, -0.166667;
-0.288675, -0.166667;
0.000000, 0.000000;
0.333333, -0.000000;
-0.166667, 0.288675;
0.166667, 0.288675;
-0.166667, -0.288675;
0.166667, -0.288675;
-0.333333, 0.000000;
0.000000, 0.000000],1,18,15);
     
% u_x-voltages
vx_pu = fi([0.000000;
0.333333;
-0.166667;
0.166667;
-0.166667;
0.166667;
-0.333333;
0.000000;
-0.288675;
0.044658;
-0.455342;
-0.122008;
-0.455342;
-0.122008;
-0.622008;
-0.288675;
0.288675;
0.622008;
0.122008;
0.455342;
0.122008;
0.455342;
-0.044658;
0.288675;
0.000000;
0.333333;
-0.166667;
0.166667;
-0.166667;
0.166667;
-0.333333;
0.000000;
-0.000000;
0.333333;
-0.166667;
0.166667;
-0.166667;
0.166667;
-0.333333;
-0.000000;
-0.288675;
0.044658;
-0.455342;
-0.122008;
-0.455342;
-0.122008;
-0.622008;
-0.288675;
0.288675;
0.622008;
0.122008;
0.455342;
0.122008;
0.455342;
-0.044658;
0.288675;
0.000000;
0.333333;
-0.166667;
0.166667;
-0.166667;
0.166667;
-0.333333;
0.000000],1,18,15);

% u_y-voltages
vy_pu = fi([0.000000;
-0.000000;
-0.288675;
-0.288675;
0.288675;
0.288675;
0.000000;
0.000000;
0.166667;
0.166667;
-0.122008;
-0.122008;
0.455342;
0.455342;
0.166667;
0.166667;
0.166667;
0.166667;
-0.122008;
-0.122008;
0.455342;
0.455342;
0.166667;
0.166667;
0.333333;
0.333333;
0.044658;
0.044658;
0.622008;
0.622008;
0.333333;
0.333333;
-0.333333;
-0.333333;
-0.622008;
-0.622008;
-0.044658;
-0.044658;
-0.333333;
-0.333333;
-0.166667;
-0.166667;
-0.455342;
-0.455342;
0.122008;
0.122008;
-0.166667;
-0.166667;
-0.166667;
-0.166667;
-0.455342;
-0.455342;
0.122008;
0.122008;
-0.166667;
-0.166667;
0.000000;
-0.000000;
-0.288675;
-0.288675;
0.288675;
0.288675;
0.000000;
0.000000],1,18,15);

pu_ud = fi(v_DC_pu * (vd_pu(index,1) * cos_angle + vd_pu(index,2) * sin_angle),1,27,24);
pu_uq = fi(v_DC_pu * (vq_pu(index,1) * -sin_angle + vq_pu(index,2) * cos_angle),1,27,24);
pu_ux = fi(v_DC_pu * vx_pu(index),1,27,24);
pu_uy = fi(v_DC_pu * vy_pu(index),1,27,24);
